simulink model "simulink_lab4_manoel"  (R2018a)
settings: Solver=VariableStepAuto  StartTime=0.0  StopTime=10.0  RelTol=1e-3
values from neighbouring files (symbols this model uses):
  atraso = stt    [manoel_outubro2.m]    (also in naao_roda.m = infor.SettlingTime; pre6_teste.m = infor.SettlingTime; pre_lab3.m = infor.SettlingTime; pre_lab3_lab.m = infor.SettlingTime)
  b0 = 18    [naao_roda.m]    (also in pre6_teste.m; pre_lab3.m; pre_lab3_2.m; pre_lab3_lab.m)
  ganho = 0.01027*infor.SettlingMax    [manoel_outubro2.m]    (also in naao_roda.m; pre6_teste.m; pre_lab3.m; pre_lab3_lab.m)
  Kpf = 1.0436    [pre_lab3.m]    (also in pre_lab3_lab.m; pre_lab4.m; pre_pedro.m = 1/dcgain(EE))
  p1 = q0*b1    [pre_lab3_2.m]    (also in pre_lab4.m; pre_lab4_2.m)
  p2 = q0*b2    [pre_lab3_2.m]    (also in pre_lab4.m; pre_lab4_2.m)
  q0 = 0.577    [naao_roda.m]    (also in pre_lab3.m; pre_lab3_2.m = 1/sum(mad.num{1}); pre_lab3_lab.m; pre_lab4.m = 1/sum(mad.num{1}))
  q1 = q0*a1    [pre_lab3_2.m]    (also in pre_lab4.m; pre_lab4_2.m)
  q2 = q0*a2    [pre_lab3_2.m]    (also in pre_lab4.m; pre_lab4_2.m)
  R0 = round(r0,1)    [naao_roda.m]    (also in pre6_teste.m; pre_lab3.m; pre_lab3_lab.m; pre_lab4.m)
  T0 = round(t0,3)    [naao_roda.m]    (also in pre6_teste.m = 0.063; pre_lab3.m; pre_lab3_2.m = 0.0640576; pre_lab3_lab.m)
  Umax = 10    [naao_roda.m]    (also in pre6_teste.m; pre_lab3.m; pre_lab3_lab.m; pre_lab4.m)
undefined symbols (not defined in the file or in its folder): p1S, p2S, q0p, q0S, q1S, q2S, T0p, T0S
settings Model: Creator=joaovitor  LastModifiedBy=joaovitor

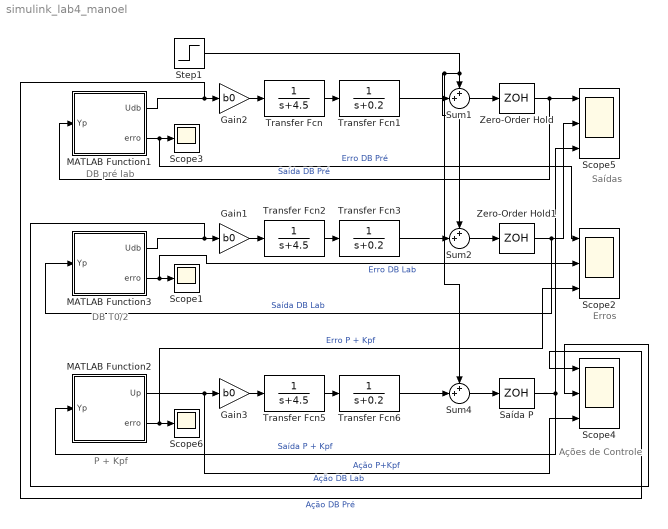
== system simulink_lab4_manoel ==
  note: Ações de Controle
  note: Erros
  note: Saídas
  note: P + Kpf
  note: DB T0/2
  note: DB pré lab
  Gain1 : Gain  Gain=b0
  Gain2 : Gain  Gain=b0
  Gain3 : Gain  Gain=b0
  MATLAB Function1 : MATLAB Function  TreatAsAtomicUnit=on
  MATLAB Function2 : MATLAB Function  TreatAsAtomicUnit=on
  MATLAB Function3 : MATLAB Function  TreatAsAtomicUnit=on
  Saída P : ZeroOrderHold  SampleTime=T0p
  Scope1 : Scope
  Scope2 : Scope  NumInputPorts=3
  Scope3 : Scope
  Scope4 : Scope  NumInputPorts=3
  Scope5 : Scope  NumInputPorts=3
  Scope6 : Scope
  Step1 : Step  Time=3*atraso  After=10*ganho  SampleTime=0
  Sum1 : Sum  Inputs=++|
  Sum2 : Sum  Inputs=++|
  Sum4 : Sum  Inputs=++|
  Transfer Fcn : TransferFcn  Denominator=[1 4.5]
  Transfer Fcn1 : TransferFcn  Denominator=[1 0.2]
  Transfer Fcn2 : TransferFcn  Denominator=[1 4.5]
  Transfer Fcn3 : TransferFcn  Denominator=[1 0.2]
  Transfer Fcn5 : TransferFcn  Denominator=[1 4.5]
  Transfer Fcn6 : TransferFcn  Denominator=[1 0.2]
  Zero-Order Hold : ZeroOrderHold  SampleTime=T0
  Zero-Order Hold1 : ZeroOrderHold  SampleTime=T0S
  wires:
  MATLAB Function1/2(erro) -> Scope2/1, Scope3/1  "Erro DB Pré"
  Transfer Fcn/1 -> Transfer Fcn1/1
  Gain2/1 -> Transfer Fcn/1
  MATLAB Function1/1(Udb) -> Scope4/1, Gain2/1  "Ação DB Pré"
  Transfer Fcn1/1 -> Sum1/2
  Transfer Fcn3/1 -> Sum2/2
  MATLAB Function3/1(Udb) -> Scope4/2, Gain1/1  "Ação DB Lab"
  Gain1/1 -> Transfer Fcn2/1
  Transfer Fcn2/1 -> Transfer Fcn3/1
  MATLAB Function3/2(erro) -> Scope2/2, Scope1/1  "Erro DB Lab"
  Sum1/1 -> Zero-Order Hold/1
  Zero-Order Hold/1 -> Scope5/1, MATLAB Function1/1(Yp)  "Saída DB Pré"
  Sum2/1 -> Zero-Order Hold1/1
  Zero-Order Hold1/1 -> Scope5/2, MATLAB Function3/1(Yp)  "Saída DB Lab"
  Step1/1 -> Sum2/1, Sum4/1, Sum1/1
  Transfer Fcn5/1 -> Transfer Fcn6/1
  Gain3/1 -> Transfer Fcn5/1
  Transfer Fcn6/1 -> Sum4/2
  MATLAB Function2/1(Up) -> Scope4/3, Gain3/1  "Ação P+Kpf"
  Sum4/1 -> Saída P/1
  Saída P/1 -> Scope5/3, MATLAB Function2/1(Yp)  "Saída P + Kpf"
  MATLAB Function2/2(erro) -> Scope2/3, Scope6/1  "Erro P + Kpf"

== matlab function simulink_lab4_manoel/MATLAB Function1 ==
  data: Yp input; q0 parameter; q1 parameter; q2 parameter; Umax parameter; p1 parameter; p2 parameter; Udb output; erro output; R0 parameter; T0 parameter
function [Udb,erro] = fcn(Yp, q0, q1, q2, Umax, p1, p2, R0, T0)    

persistent u0;
persistent u00;
persistent e0;
persistent e00;

if isempty(u0)
    u0=0;
    u00=0;
    e0=0;
    e00=0;
end

% GDB = tf([q0 q1 q2],[1 -p1 -p2],T0);

erro=R0-Yp;

Udb=q0*erro+q1*e0+q2*e00+p1*u0+p2*u00;

e00=e0;
e0=erro;
u00=u0;
u0=Udb;

if(abs(Udb)>Umax)
    Udb=Umax*sign(Udb)
end

== matlab function simulink_lab4_manoel/MATLAB Function3 ==
  data: Yp input; q0S parameter; q1S parameter; q2S parameter; Umax parameter; p1S parameter; p2S parameter; Udb output; erro output; R0 parameter
function [Udb,erro] = fcn(Yp, q0S, q1S, q2S, Umax, p1S, p2S, R0)    

persistent u0;
persistent u00;
persistent e0;
persistent e00;

if isempty(u0)
    u0=0;
    u00=0;
    e0=0;
    e00=0;
end

% GDB = tf([q0 q1 q2],[1 -p1 -p2],T0);

erro=R0-Yp;

Udb=q0S*erro+q1S*e0+q2S*e00+p1S*u0+p2S*u00;

e00=e0;
e0=erro;
u00=u0
u0=Udb

if(abs(Udb)>Umax)
    Udb=Umax*sign(Udb)
end

== matlab function simulink_lab4_manoel/MATLAB Function2 ==
  data: Up output; Yp input; erro output; R0 parameter; q0p parameter; Umax parameter; Kpf parameter
function [Up,erro] = fcn(Yp, R0, q0p, Umax, Kpf)    

Up=(R0*Kpf-Yp)*1.14

erro=(R0-Yp)

if(abs(Up)>Umax)
    Up=Umax*sign(Up)

Yp=Up
end
